simulink model "Sensor_Complimantary2"  (R2021a)
settings: Solver=FixedStepAuto  StartTime=0.0  StopTime=Inf  RelTol=1e-3  EnableMultiTasking=on
libraries: arduinosensorlib x1
settings Model: SILPILModeSetting=veronly  ExtModeTrigDuration=2  Creator=Samsung  LastModifiedBy=user
settings OptimizationCC: EnhancedBackFolding=on  PassReuseOutputArgsAs=Individual arguments  ZeroExternalMemoryAtStartup=off  ZeroInternalMemoryAtStartup=off  MaxStackSize=64  OptimizeBlockOrder=speed  DifferentSizesBufferReuse=on  OptimizationCustomize=off  EfficientTunableParamExpr=on
settings DebuggingCC: ParameterTunabilityLossMsg=error
settings HardwareCC: ProdBitPerInt=16  ProdBitPerPointer=16  ProdBitPerSizeT=16  ProdBitPerPtrDiffT=16  ProdLargestAtomicFloat=None  ProdWordSize=8  ProdHWDeviceType=Atmel->AVR
settings SFSimCC: MATLABDynamicMemAlloc=off
settings RTWCC: SystemTargetFile=ert.tlc  HardwareBoard=Arduino Uno  TemplateMakefile=ert_default_tmf  Toolchain=Arduino AVR  BuildConfiguration=Faster Runs
settings CodeAppCC: ForceParamTrailComments=on  IgnoreCustomStorageClasses=off  OperatorAnnotations=on  SimulinkDataObjDesc=on  SFDataObjDesc=on  InsertBlockDesc=on
settings ERTTargetCC: SupportContinuousTime=on  SupportVariableSizeSignals=on  ExtModeStaticAllocSize=250

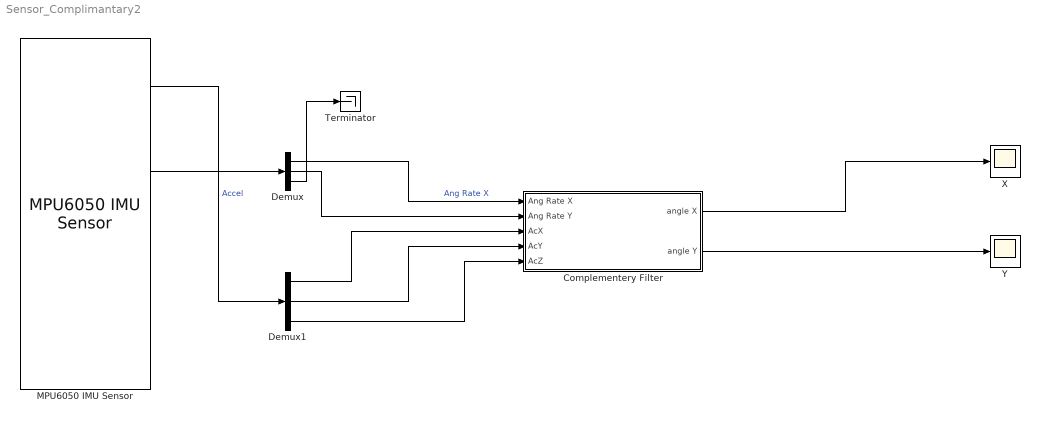
== system Sensor_Complimantary2 ==
  Complementery Filter : Subsystem
  Demux : Demux  Outputs=3
  Demux1 : Demux  Outputs=3
  MPU6050 IMU Sensor : arduinosensorlib/MPU6050 IMU Sensor  SlaveAddress=0x68  Accel=on  AngularRate=on  Temperature=on  Status=on  EulerAngles=off  Quat=off  AccelRange=2G  GyroRange=250 dps  DmpOdr=200 Hz  Dlpf=Accelerometer: 260Hz, Gyroscope: 256Hz  SampleTime=-1
      settings: SourceProductBaseCode=ARDUINO
  Terminator : Terminator
  X : Scope
  Y : Scope
  wires:
  MPU6050 IMU Sensor/2 -> Demux/1
  MPU6050 IMU Sensor/1 -> Demux1/1  "Accel"
  Demux/1 -> Complementery Filter/1(Ang Rate X)  "Ang Rate X"
  Demux1/1 -> Complementery Filter/3(AcX)
  Demux1/2 -> Complementery Filter/4(AcY)
  Demux1/3 -> Complementery Filter/5(AcZ)
  Complementery Filter/1(angle X) -> X/1
  Demux/2 -> Complementery Filter/2(Ang Rate Y)
  Complementery Filter/2(angle Y) -> Y/1
  Demux/3 -> Terminator/1

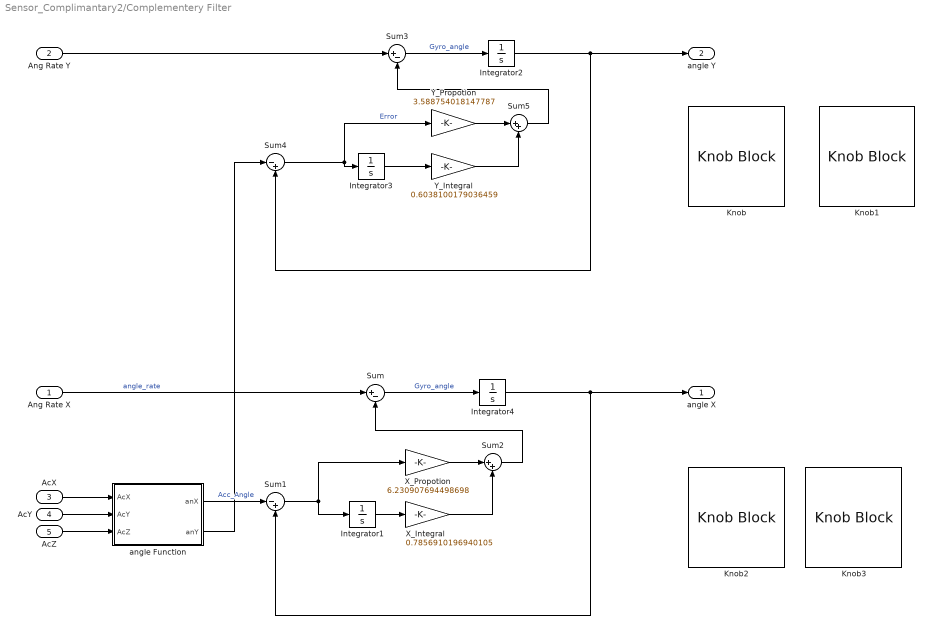
== system Sensor_Complimantary2/Complementery Filter ==
  Ang Rate X : Inport
  Ang Rate Y : Inport  Port=2
  AcX : Inport  Port=3
  AcY : Inport  Port=4
  AcZ : Inport  Port=5
  Integrator{1..4} (4 alike) : Integrator
  Knob : KnobBlock  ScaleMin=3  ScaleMax=4
  Knob1 : KnobBlock  ScaleMax=1
  Knob2 : KnobBlock  ScaleMax=10
  Knob3 : KnobBlock  ScaleMax=1
  Sum : Sum  Inputs=|+-
  Sum1 : Sum  Inputs=|-+
  Sum2 : Sum  Inputs=|++
  Sum3 : Sum  Inputs=|+-
  Sum4 : Sum  Inputs=|-+
  Sum5 : Sum  Inputs=|++
  X_Integral : Gain  Gain=0.7856910196940105
  X_Propotion : Gain  Gain=6.230907694498698
  Y_Integral : Gain  Gain=0.6038100179036459
  Y_Propotion : Gain  Gain=3.588754018147787
  angle Function : MATLAB Function  TreatAsAtomicUnit=on
  angle X : Outport
  angle Y : Outport  Port=2
  wires:
  X_Integral/1 -> Sum2/2
  Sum/1 -> Integrator4/1  "Gyro_angle"
  Ang Rate X/1 -> Sum/1  "angle_rate"
  Integrator1/1 -> X_Integral/1
  X_Propotion/1 -> Sum2/1
  AcY/1 -> angle Function/2(AcY)
  Sum1/1 -> X_Propotion/1, Integrator1/1
  Sum2/1 -> Sum/2
  angle Function/1(anX) -> Sum1/1  "Acc_Angle"
  AcX/1 -> angle Function/1(AcX)
  AcZ/1 -> angle Function/3(AcZ)
  Integrator3/1 -> Y_Integral/1
  Y_Propotion/1 -> Sum5/1
  Y_Integral/1 -> Sum5/2
  Sum3/1 -> Integrator2/1  "Gyro_angle"
  Sum5/1 -> Sum3/2
  Sum4/1 -> Integrator3/1, Y_Propotion/1  "Error"
  Ang Rate Y/1 -> Sum3/1
  angle Function/2(anY) -> Sum4/1
  Integrator2/1 -> angle Y/1, Sum4/2
  Integrator4/1 -> angle X/1, Sum1/2

== matlab function Sensor_Complimantary2/Complementery Filter/angle Function ==
  data: AcX input; anX output; AcY input; AcZ input; anY output
function [anX,anY] = fcn(AcX,AcY,AcZ)

anX = atan(-AcY / (sqrt(AcX^2 + AcZ^2))) * 180/pi;
anY = atan(-AcX / (sqrt(AcY^2 + AcZ^2))) * 180/pi;

end
